simulink model "dorrsystem"  (R2020b)
settings: Solver=FixedStepAuto  StartTime=0.0  StopTime=10  FixedStep=1  RelTol=1e-3
libraries: simulink x1
settings Model: Creator=99003736  LastModifiedBy=99003736

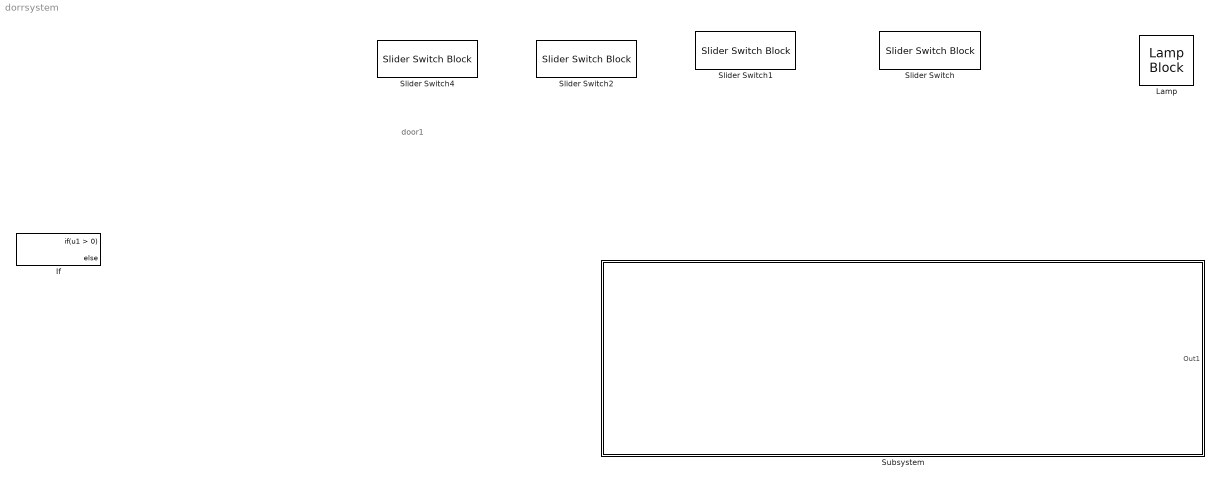
== system dorrsystem ==
  note: door1
  If : If
  Lamp : LampBlock
  Slider Switch{,1..2,4} (4 alike) : SliderSwitchBlock
      settings: Values={{'Off', 'On'}, [0 1]}
  Subsystem : Subsystem

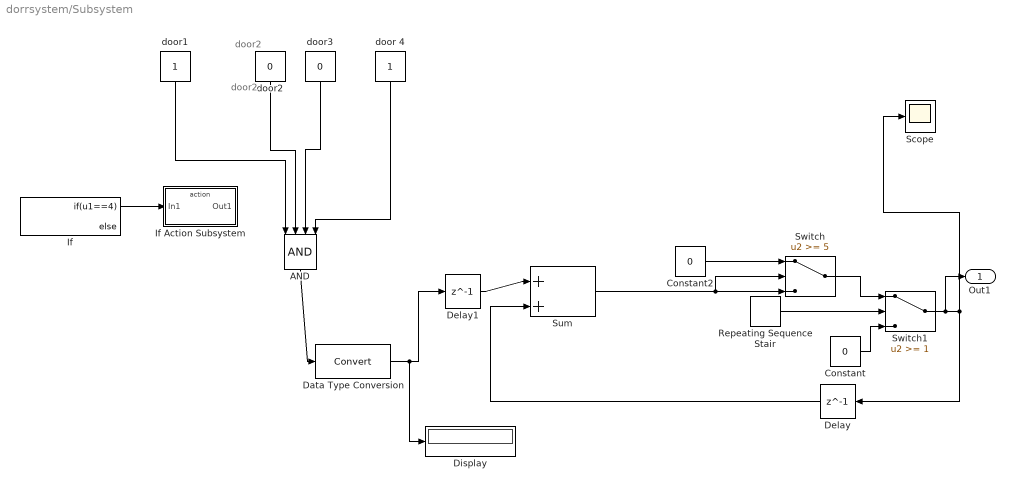
== system dorrsystem/Subsystem ==
  note: door2
  note: door2
  AND : Logic  Inputs=4  IconShape=distinctive  AllPortsSameDT=off  OutDataTypeStr=boolean
  Constant : Constant  Value=0
  Constant2 : Constant  Value=0
  Data Type Conversion : DataTypeConversion
  Delay : Delay  DelayLength=1
  Delay1 : Delay  DelayLength=1
  Display : Display
  If : If  IfExpression=u1==4
  If Action Subsystem : Subsystem  TreatAsAtomicUnit=on
  Repeating Sequence Stair : simulink/Sources/Repeating Sequence Stair  OutValues=[1 1]  tsamp=-1  OutMin=[]  OutMax=[]  OutDataTypeStr=double  OutputDataTypeScalingMode=double  OutDataType=fixdt(0,8)  ConRadixGroup=Best Precision: Vector-wise  OutScaling=2^-12
  Scope : Scope
  Sum : Sum  Inputs=|++
  Switch : Switch  Threshold=5
  Switch1 : Switch  Threshold=1
  door 4 : Constant
  door1 : Constant
  door2 : Constant  Value=0
  door3 : Constant  Value=0
  Out1 : Outport
  wires:
  Delay/1 -> Sum/2
  Data Type Conversion/1 -> Display/1, Delay1/1
  Sum/1 -> Switch/2, Switch/3
  door1/1 -> AND/1
  Constant2/1 -> Switch/1
  door3/1 -> AND/3
  Delay1/1 -> Sum/1
  door2/1 -> AND/2
  door 4/1 -> AND/4
  AND/1 -> Data Type Conversion/1
  Switch/1 -> Switch1/1
  Constant/1 -> Switch1/3
  Repeating Sequence Stair/1 -> Switch1/2
  Switch1/1 -> Out1/1, Delay/1, Scope/1
  If/1 -> If Action Subsystem/1(In1)

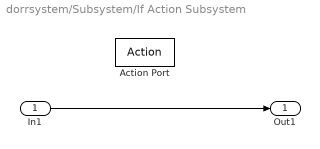
== system dorrsystem/Subsystem/If Action Subsystem ==
  In1 : Inport
  Action Port : ActionPort
  Out1 : Outport
  wires:
  In1/1 -> Out1/1
